simulink model "PointProcessSimulationThinning"  (Simulink 7.7)
settings: Solver=FixedStepDiscrete  SolverMode=SingleTasking  StartTime=0.0  StopTime=10  FixedStep=Ts  RelTol=1e-3
values from neighbouring files (symbols this model uses):
  mu = b    [Analysis.m]    (also in Covariate.m = mean(covObj); nstColl.m = bVals)
  simTypeSelect = 0    [CIF.m]
  Ts = hist.Ts    [CIF.m]
undefined symbols (not defined in the file or in its folder): DiscIntNeverNeededParam, TsInt
libraries: cstblocks x3, simulink x2, dspsigops x2
settings Model: Creator=Developer  LastModifiedBy=Developer  SimulationMode=accelerator
settings DataIOCC: LimitDataPoints=off  LoadExternalInput=on  SaveFormat=StructureWithTime  SaveOutput=off  SaveTime=off

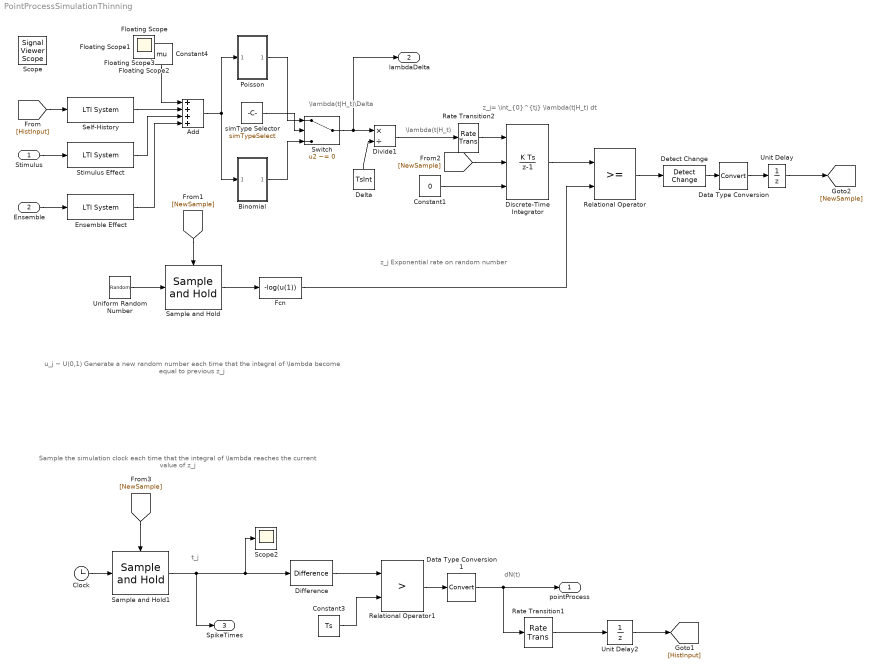
== system PointProcessSimulationThinning ==
  note: u_j ~ U(0,1)
      | Generate a new random number
      | each time that the integral of \lambda
      | become equal to previous z_j
  note: z_j
      | Exponential rate on random number
  note: z_j= \int_{0}^{tj} \lambda(t|H_t) dt
  note: dN(t)
  note: \lambda(t|H_t)
  note: \lambda(t|H_t)\Delta
  note: t_j
  note: Sample the simulation clock each time that the
      | integral of \lambda reaches the current value of z_j
  Stimulus : Inport
  Ensemble : Inport  Port=2
  Add : Sum  Inputs=++++
  Binomial : Subsystem
  Clock : Clock
      settings: Decimation=10
  Constant1 : Constant  Value=0
  Constant3 : Constant  Value=Ts  SampleTime=Ts
  Constant4 : Constant  Value=mu
  Data Type Conversion : DataTypeConversion
  Data Type Conversion1 : DataTypeConversion
  Delta : Constant  Value=TsInt
  Detect Change : simulink/Logic and Bit Operations/Detect Change  SystemSampleTime=-1  vinit=0
  Difference : simulink/Discrete/Difference  SystemSampleTime=-1  ICPrevInput=0.0  OutMin=[]  OutMax=[]  OutDataType=fixdt(1, 16)  OutScaling=2^-10  DoSatur=off
  Discrete-Time Integrator : DiscreteIntegrator  ExternalReset=either  InitialConditionSource=external  SampleTime=Ts  ICPrevOutput=DiscIntNeverNeededParam  ICPrevScaledInput=DiscIntNeverNeededParam
  Divide1 : Product  Inputs=*/  SampleTime=TsInt
  Ensemble Effect : cstblocks/LTI System  SystemSampleTime=-1  sys=E  IC=[]
  Fcn : Fcn  Expr=-log(u(1))
  Poisson : Subsystem
  Rate Transition1 : RateTransition  OutPortSampleTime=TsInt
  Rate Transition2 : RateTransition  OutPortSampleTime=Ts
  Relational Operator : RelationalOperator  SampleTime=Ts
  Relational Operator1 : RelationalOperator  Operator=>
  Sample and Hold : dspsigops/Sample and Hold  SystemSampleTime=-1  trig=Rising edge  initCond=rand(1,1)  latchinput=on
  Sample and Hold1 : dspsigops/Sample and Hold  SystemSampleTime=-1  trig=Rising edge  initCond=0  latchinput=on
  Scope2 : Scope
      settings: YMin=1.05  YMax=1.25
  Self-History : cstblocks/LTI System  SystemSampleTime=-1  sys=H  IC=[]
  Stimulus Effect : cstblocks/LTI System  SystemSampleTime=-1  sys=S  IC=[]
  Switch : Switch  Criteria=u2 ~= 0
  Uniform Random Number : UniformRandomNumber  Minimum=0  SampleTime=Ts
  Unit Delay : UnitDelay  SampleTime=Ts
  Unit Delay2 : UnitDelay  SampleTime=-1
  simType Selector : Constant  Value=simTypeSelect
  pointProcess : Outport
  lambdaDelta : Outport  Port=2
  SpikeTimes : Outport  Port=3
  Floating Scope{,1..3} (4 alike) : Scope
      Floating Scope settings: Floating=on  YMin=25  YMax=275  SaveName=ScopeData2
      Floating Scope1 settings: Floating=on  SaveName=ScopeData3
      Floating Scope2 settings: Floating=on  YMin=1  YMax=1  SaveName=ScopeData4
      Floating Scope3 settings: Floating=on  SaveName=ScopeData5
  Scope : SignalViewerScope  IOType=viewer  RefreshTime=0.035000
      settings: YMin=-1  YMax=1
  wires:
  Uniform Random Number/1 -> Sample and Hold/1
  Sample and Hold/1 -> Fcn/1
  Relational Operator/1 -> Detect Change/1
  Fcn/1 -> Relational Operator/2
  Detect Change/1 -> Data Type Conversion/1
  Data Type Conversion/1 -> Unit Delay/1
  Constant4/1 -> Add/1
  Self-History/1 -> Add/2
  Stimulus Effect/1 -> Add/3
  Add/1 -> Binomial/1(In1), Poisson/1(In1)
  Ensemble Effect/1 -> Add/4
  Delta/1 -> Divide1/2
  Divide1/1 -> Rate Transition2/1
  Binomial/1(Out1) -> Switch/3
  Switch/1 -> Divide1/1, lambdaDelta/1
  Poisson/1(Out1) -> Switch/1
  simType Selector/1 -> Switch/2
  Stimulus/1 -> Stimulus Effect/1
  Unit Delay/1 -> [NewSample]
  Discrete-Time Integrator/1 -> Relational Operator/1
  Constant1/1 -> Discrete-Time Integrator/3
  Rate Transition2/1 -> Discrete-Time Integrator/1
  Ensemble/1 -> Ensemble Effect/1
  [HistInput] -> Self-History/1
  [NewSample] -> Sample and Hold/Trigger
  [NewSample] -> Discrete-Time Integrator/2
  Clock/1 -> Sample and Hold1/1
  Sample and Hold1/1 -> Scope2/1, Difference/1, SpikeTimes/1
  [NewSample] -> Sample and Hold1/Trigger
  Difference/1 -> Relational Operator1/1
  Constant3/1 -> Relational Operator1/2
  Relational Operator1/1 -> Data Type Conversion1/1
  Data Type Conversion1/1 -> pointProcess/1, Rate Transition1/1
  Rate Transition1/1 -> Unit Delay2/1
  Unit Delay2/1 -> [HistInput]

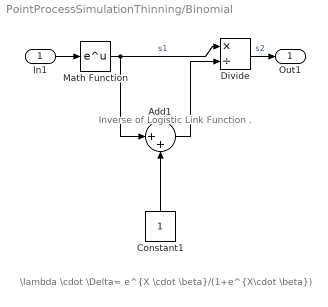
== system PointProcessSimulationThinning/Binomial ==
  note: Inverse of Logistic Link Function
      |
      |
      |
      |
      |
      |
      |
      |
      |
      |
      | .
  note: \lambda \cdot \Delta= e^{X \cdot \beta}/(1+e^{X\cdot \beta})
  In1 : Inport
  Add1 : Sum  Inputs=|++
  Constant1 : Constant
  Divide : Product  Inputs=*/
  Math Function : Math  SaturateOnIntegerOverflow=on
  Out1 : Outport
  wires:
  Constant1/1 -> Add1/2
  Math Function/1 -> Add1/1, Divide/1  "s1"
  Add1/1 -> Divide/2
  Divide/1 -> Out1/1  "s2"
  In1/1 -> Math Function/1

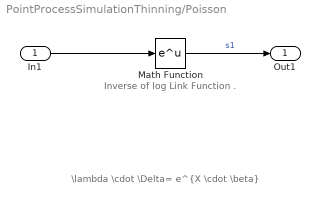
== system PointProcessSimulationThinning/Poisson ==
  note: \lambda \cdot \Delta= e^{X \cdot \beta}
  note: Inverse of log Link Function
      |
      |
      |
      |
      |
      |
      | .
  In1 : Inport
  Math Function : Math  SaturateOnIntegerOverflow=on
  Out1 : Outport
  wires:
  In1/1 -> Math Function/1
  Math Function/1 -> Out1/1  "s1"
